simulink model "model2"  (R2021b)
settings: Solver=ode45  StartTime=0.0  StopTime=20.0  MaxStep=0.01  RelTol=1e-3
settings Model: Creator=Studenci  LastModifiedBy=Studenci

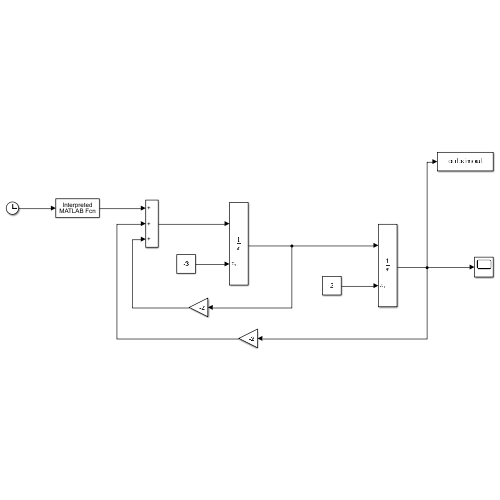
[thumbnail: Simulink's stored preview of the top-level diagram]
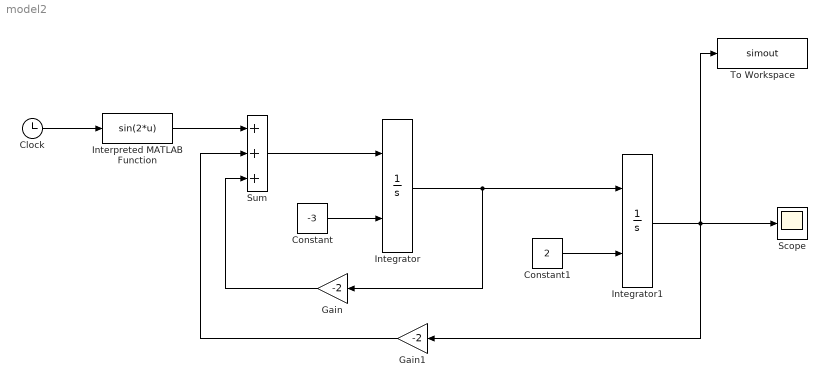
== system model2 ==
  Clock : Clock
  Constant : Constant  Value=-3
  Constant1 : Constant  Value=2
  Gain : Gain  Gain=-2
  Gain1 : Gain  Gain=-2
  Integrator : Integrator  InitialConditionSource=external
  Integrator1 : Integrator  InitialConditionSource=external
  Interpreted MATLAB Function : MATLABFcn  MATLABFcn=sin(2*u)
  Scope : Scope
  Sum : Sum  Inputs=+++
  To Workspace : ToWorkspace  VariableName=simout  SaveFormat=Timeseries  SampleTime=-1
  wires:
  Constant/1 -> Integrator/2
  Integrator/1 -> Integrator1/1, Gain/1
  Sum/1 -> Integrator/1
  Clock/1 -> Interpreted MATLAB Function/1
  Gain/1 -> Sum/3
  Interpreted MATLAB Function/1 -> Sum/1
  Constant1/1 -> Integrator1/2
  Integrator1/1 -> To Workspace/1, Scope/1, Gain1/1
  Gain1/1 -> Sum/2
